simulink model "_Simulink_DualBoxcarAveragerFixedPoint"  (R2023b)
settings: Solver=FixedStepDiscrete  StartTime=0.0  StopTime=0.001  RelTol=1e-3
model workspace (MAT data in the model file):
  test = 0
undefined symbols (not defined in the file): a, b, c
libraries: hdlsllib x3, simulink x2, dspsrcs4 x1
settings Model: DataTypeOverride=Off  FPTShortcutValueString='{{},{''BaselineRun'',1,1,1,''BaselineRun'','''',{},''M'',''F'',''''},{''EmbeddedRun'',1,1,1,''EmbeddedRun'','''',{},''M'','''',''''},{''BaselineRun_5'',1,1,1,''BaselineRun_5'','''',{},''M'',''F'',''''}}'  Creator=max_d  LastModifiedBy=heyan
settings SolverCC: AlgebraicLoopSolver=TrustRegion  AutoInsertRateTranBlk=on
settings DataIOCC: LimitDataPoints=on  SaveOutput=off  SaveTime=off
settings OptimizationCC: BlockReduction=off  ConditionallyExecuteInputs=off  DefaultParameterBehavior=Inlined  InheritOutputTypeSmallerThanSingle=on  LifeSpan=inf
settings DebuggingCC: SignalRangeChecking=warning  AlgebraicLoopMsg=error  SingleTaskRateTransMsg=error  UnconnectedInputMsg=warning  UnconnectedOutputMsg=warning  UnconnectedLineMsg=warning  AllowSymbolicDim=off  StrictBusMsg=ErrorOnBusTreatedAsVector  SFUnexpectedBacktrackingDiag=warning  SFNoUnconditionalDefaultTransitionDiag=warning  SFExecutionAtInitializationDiag=none  ArithmeticOperatorsInVariantConditions=warning
settings HardwareCC: ProdBitPerPointer=32  ProdBitPerSizeT=32  ProdBitPerPtrDiffT=32  ProdLargestAtomicFloat=None  ProdIntDivRoundTo=Undefined  ProdEndianess=Unspecified  ProdWordSize=32  ProdHWDeviceType=ASIC/FPGA->ASIC/FPGA  ProdEqTarget=off
settings ModelReferenceCC: EnableRefExpFcnMdlSchedulingChecks=on
settings SFSimCC: SimUseLocalCustomCode=off  CustomCodeUndefinedFunction=UseInterfaceOnly
settings RTWCC: RTWUseLocalCustomCode=off  DLArmComputeVersion=19.05
settings CodeAppCC: StateflowObjectComments=on
settings GRTTargetCC: TargetLangStandard=C89/C90 (ANSI)
settings ConfigComp: CovScope=ReferencedModels  CovMetricSettings=dw  CovSaveCumulativeToWorkspaceVar=on  CovSaveSingleToWorkspaceVar=on  CovExternalEMLEnable=off  CovSFcnEnable=off

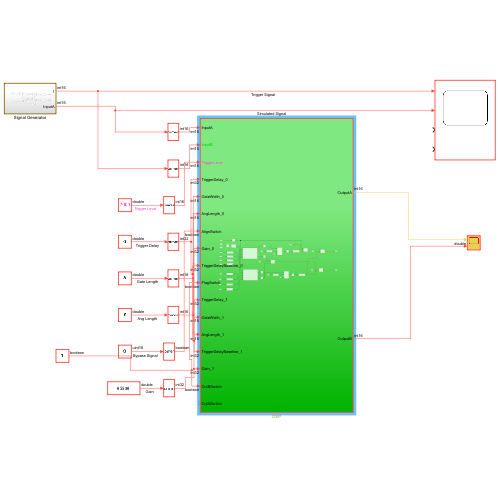
[thumbnail: Simulink's stored preview of the top-level diagram]
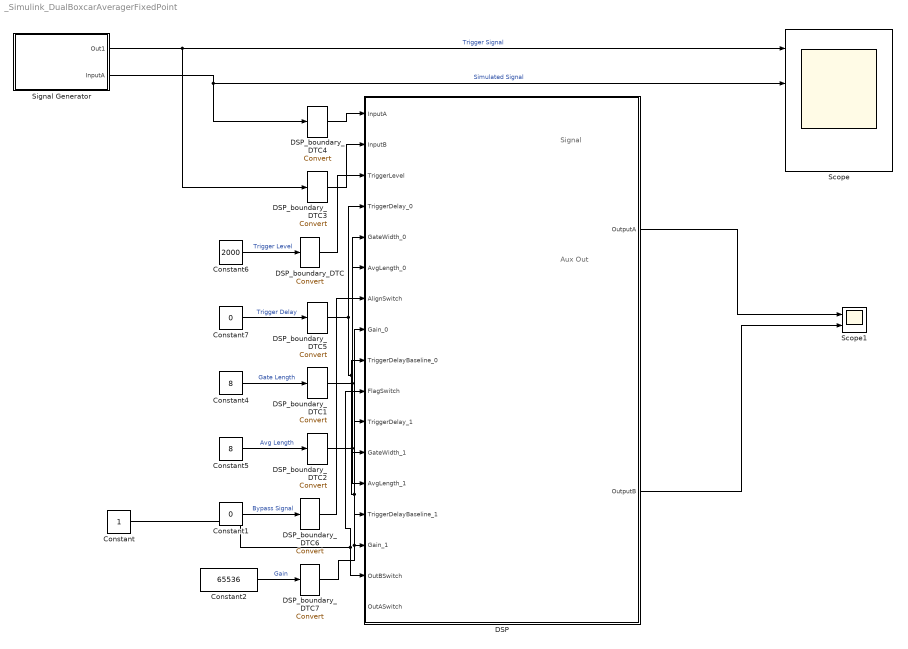
== system _Simulink_DualBoxcarAveragerFixedPoint ==
  note: Signal
  note: Aux Out
  Constant : Constant  OutDataTypeStr=boolean  SampleTime=1/312.5e6
  Constant1 : Constant  Value=0  OutDataTypeStr=fixdt(0,16,0)  SampleTime=1/312.5e6
  Constant2 : Constant  Value=65536  OutDataTypeStr=double  SampleTime=1/312.5e6
  Constant4 : Constant  Value=8  OutDataTypeStr=double  SampleTime=1/312.5e6
  Constant5 : Constant  Value=8  OutDataTypeStr=double  SampleTime=1/312.5e6
  Constant6 : Constant  Value=2000  OutDataTypeStr=double  SampleTime=1/312.5e6
  Constant7 : Constant  Value=0  OutDataTypeStr=double  SampleTime=1/312.5e6
  DSP : Subsystem
  DSP_boundary_DTC{,1..7} (8 alike) : DataTypeConversion
  Scope : Scope  NumInputPorts=4
  Scope1 : Scope  NumInputPorts=2
  Signal Generator : Subsystem
  wires:
  Constant2/1 -> DSP_boundary_DTC7/1  "Gain"
  Constant1/1 -> DSP_boundary_DTC6/1  "Bypass Signal"
  Constant5/1 -> DSP_boundary_DTC2/1  "Avg Length"
  Constant4/1 -> DSP_boundary_DTC1/1  "Gate Length"
  Constant7/1 -> DSP_boundary_DTC5/1  "Trigger Delay"
  Constant6/1 -> DSP_boundary_DTC/1  "Trigger Level"
  Signal Generator/1(Out1) -> DSP_boundary_DTC3/1, Scope/1  "Trigger Signal"
  Signal Generator/2(InputA) -> DSP_boundary_DTC4/1, Scope/2  "Simulated Signal"
  DSP_boundary_DTC/1 -> DSP/3(TriggerLevel)
  DSP_boundary_DTC1/1 -> DSP/12(GateWidth_1), DSP/5(GateWidth_0)
  DSP_boundary_DTC2/1 -> DSP/13(AvgLength_1), DSP/6(AvgLength_0)
  DSP_boundary_DTC3/1 -> DSP/2(InputB)
  DSP_boundary_DTC4/1 -> DSP/1(InputA)
  DSP_boundary_DTC5/1 -> DSP/9(TriggerDelayBaseline_0), DSP/14(TriggerDelayBaseline_1), DSP/11(TriggerDelay_1), DSP/4(TriggerDelay_0)
  DSP_boundary_DTC7/1 -> DSP/15(Gain_1), DSP/8(Gain_0)
  DSP_boundary_DTC6/1 -> DSP/7(AlignSwitch)
  Constant/1 -> DSP/16(OutBSwitch), DSP/10(FlagSwitch)
  DSP/1(OutputA) -> Scope1/1
  DSP/2(OutputB) -> Scope1/2

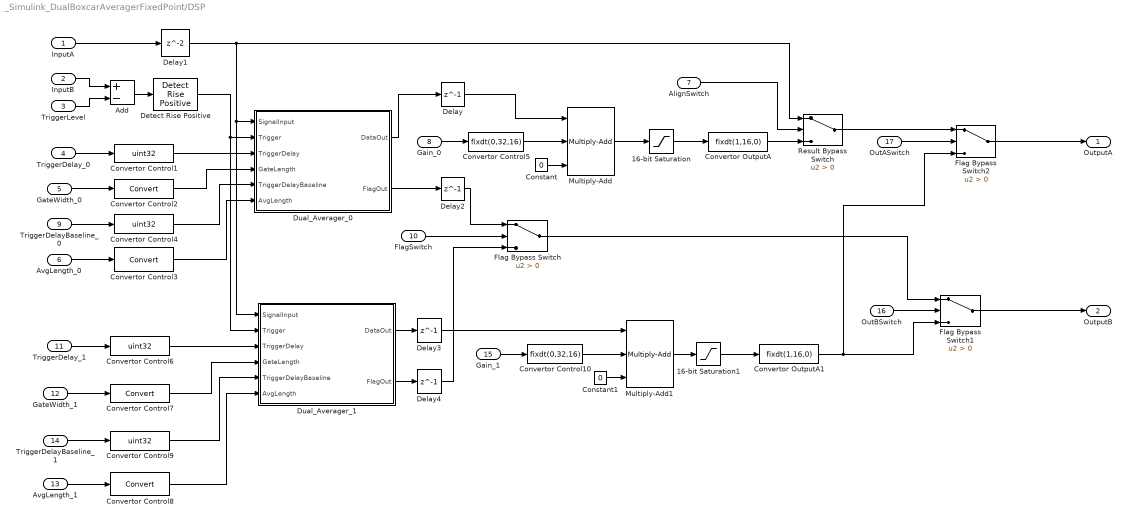
== system _Simulink_DualBoxcarAveragerFixedPoint/DSP ==
  InputA : Inport  OutDataTypeStr=fixdt(1,16,0)
  InputB : Inport  Port=2  OutDataTypeStr=fixdt(1,16,0)
  TriggerLevel : Inport  Port=3  OutDataTypeStr=fixdt(1,16,0)
  TriggerDelay_0 : Inport  Port=4  OutDataTypeStr=fixdt(1,32,0)
  GateWidth_0 : Inport  Port=5  OutDataTypeStr=fixdt(1,16,0)
  AvgLength_0 : Inport  Port=6  OutDataTypeStr=fixdt(1,16,0)
  AlignSwitch : Inport  Port=7  OutDataTypeStr=boolean
  Gain_0 : Inport  Port=8  OutDataTypeStr=fixdt(1,32,0)
  TriggerDelayBaseline_0 : Inport  Port=9  OutDataTypeStr=fixdt(1,32,0)
  FlagSwitch : Inport  Port=10  OutDataTypeStr=boolean
  TriggerDelay_1 : Inport  Port=11  OutDataTypeStr=fixdt(1,32,0)
  GateWidth_1 : Inport  Port=12  OutDataTypeStr=fixdt(1,16,0)
  AvgLength_1 : Inport  Port=13  OutDataTypeStr=fixdt(1,16,0)
  TriggerDelayBaseline_1 : Inport  Port=14  OutDataTypeStr=fixdt(1,32,0)
  Gain_1 : Inport  Port=15  OutDataTypeStr=fixdt(1,32,0)
  OutBSwitch : Inport  Port=16  OutDataTypeStr=boolean
  OutASwitch : Inport  Port=17  OutDataTypeStr=boolean
  16-bit Saturation : Saturate  UpperLimit=32767  LowerLimit=-32768
  16-bit Saturation1 : Saturate  UpperLimit=32767  LowerLimit=-32768
  Add : Sum  Inputs=+-  OutDataTypeStr=fixdt(1,17,0)
  Constant : Constant  Value=0  OutDataTypeStr=fixdt(0,1,0)  SampleTime=1/312.5e6
  Constant1 : Constant  Value=0  OutDataTypeStr=fixdt(0,1,0)  SampleTime=1/312.5e6
  Convertor Control{1,4,6,9} (4 alike) : DataTypeConversion  OutDataTypeStr=uint32  ConvertRealWorld=Stored Integer (SI)  SaturateOnIntegerOverflow=off  RndMeth=Floor
  Convertor Control10 : DataTypeConversion  OutDataTypeStr=fixdt(0,32,16)  ConvertRealWorld=Stored Integer (SI)  SaturateOnIntegerOverflow=off  RndMeth=Floor
  Convertor Control{2..3,7..8} (4 alike) : DataTypeConversion  ConvertRealWorld=Stored Integer (SI)  SaturateOnIntegerOverflow=off  RndMeth=Floor
  Convertor Control5 : DataTypeConversion  OutDataTypeStr=fixdt(0,32,16)  ConvertRealWorld=Stored Integer (SI)  SaturateOnIntegerOverflow=off  RndMeth=Floor
  Convertor OutputA : DataTypeConversion  OutDataTypeStr=fixdt(1,16,0)  SaturateOnIntegerOverflow=off  RndMeth=Floor
  Convertor OutputA1 : DataTypeConversion  OutDataTypeStr=fixdt(1,16,0)  SaturateOnIntegerOverflow=off  RndMeth=Floor
  Delay{,2..4} (4 alike) : Delay  DelayLength=1  InitialCondition=0  UseCircularBuffer=on
  Delay1 : Delay  InitialCondition=0
  Detect Rise Positive : hdlsllib/Logic and Bit Operations/Detect Rise Positive  vinit=0  OutDataTypeStr=boolean
  Dual_Averager_0 : Subsystem
  Dual_Averager_1 : Subsystem
  Flag Bypass Switch : Switch  Criteria=u2 > Threshold  SaturateOnIntegerOverflow=off  InputSameDT=off  OutDataTypeStr=Inherit: Same as first input
  Flag Bypass Switch1 : Switch  Criteria=u2 > Threshold  SaturateOnIntegerOverflow=off  InputSameDT=off  OutDataTypeStr=Inherit: Same as first input
  Flag Bypass Switch2 : Switch  Criteria=u2 > Threshold  SaturateOnIntegerOverflow=off  InputSameDT=off  OutDataTypeStr=Inherit: Same as first input
  Multiply-Add : hdlsllib/HDL Operations/Multiply-Add  Function=c+(a.*b)  datatype=Inherit: Inherit via internal rule  DoSatur=on  FMA=off
  Multiply-Add1 : hdlsllib/HDL Operations/Multiply-Add  Function=c+(a.*b)  datatype=Inherit: Inherit via internal rule  DoSatur=on  FMA=off
  Result Bypass Switch : Switch  Criteria=u2 > Threshold  OutDataTypeStr=fixdt(1,16,0)  SaturateOnIntegerOverflow=off  InputSameDT=off
  OutputA : Outport  OutDataTypeStr=fixdt(1,16,0)  VectorParamsAs1DForOutWhenUnconnected=off
  OutputB : Outport  Port=2  OutDataTypeStr=fixdt(1,16,0)  VectorParamsAs1DForOutWhenUnconnected=off
  wires:
  GateWidth_0/1 -> Convertor Control2/1
  Convertor OutputA/1 -> Result Bypass Switch/3
  Multiply-Add/1 -> 16-bit Saturation/1
  Constant/1 -> Multiply-Add/3
  TriggerLevel/1 -> Add/2
  Add/1 -> Detect Rise Positive/1
  Flag Bypass Switch/1 -> Flag Bypass Switch1/1
  16-bit Saturation/1 -> Convertor OutputA/1
  Gain_0/1 -> Convertor Control5/1
  Result Bypass Switch/1 -> Flag Bypass Switch2/1
  Convertor Control5/1 -> Multiply-Add/2
  InputA/1 -> Delay1/1
  AvgLength_0/1 -> Convertor Control3/1
  TriggerDelay_0/1 -> Convertor Control1/1
  InputB/1 -> Add/1
  TriggerDelayBaseline_0/1 -> Convertor Control4/1
  AlignSwitch/1 -> Result Bypass Switch/2
  FlagSwitch/1 -> Flag Bypass Switch/2
  TriggerDelay_1/1 -> Convertor Control6/1
  AvgLength_1/1 -> Convertor Control8/1
  GateWidth_1/1 -> Convertor Control7/1
  TriggerDelayBaseline_1/1 -> Convertor Control9/1
  Constant1/1 -> Multiply-Add1/3
  Multiply-Add1/1 -> 16-bit Saturation1/1
  Convertor Control10/1 -> Multiply-Add1/2
  16-bit Saturation1/1 -> Convertor OutputA1/1
  Gain_1/1 -> Convertor Control10/1
  OutBSwitch/1 -> Flag Bypass Switch1/2
  Convertor OutputA1/1 -> Flag Bypass Switch2/3, Flag Bypass Switch1/3
  Detect Rise Positive/1 -> Dual_Averager_1/2(Trigger), Dual_Averager_0/2(Trigger)
  Delay1/1 -> Dual_Averager_1/1(SignalInput), Dual_Averager_0/1(SignalInput), Result Bypass Switch/1
  Convertor Control1/1 -> Dual_Averager_0/3(TriggerDelay)
  Convertor Control4/1 -> Dual_Averager_0/5(TriggerDelayBaseline)
  Convertor Control2/1 -> Dual_Averager_0/4(GateLength)
  Convertor Control3/1 -> Dual_Averager_0/6(AvgLength)
  Dual_Averager_0/1(DataOut) -> Delay/1
  Dual_Averager_0/2(FlagOut) -> Delay2/1
  Convertor Control6/1 -> Dual_Averager_1/3(TriggerDelay)
  Convertor Control7/1 -> Dual_Averager_1/4(GateLength)
  Convertor Control9/1 -> Dual_Averager_1/5(TriggerDelayBaseline)
  Convertor Control8/1 -> Dual_Averager_1/6(AvgLength)
  Dual_Averager_1/2(FlagOut) -> Delay4/1
  Dual_Averager_1/1(DataOut) -> Delay3/1
  OutASwitch/1 -> Flag Bypass Switch2/2
  Flag Bypass Switch2/1 -> OutputA/1
  Flag Bypass Switch1/1 -> OutputB/1
  Delay/1 -> Multiply-Add/1
  Delay2/1 -> Flag Bypass Switch/1
  Delay3/1 -> Multiply-Add1/1
  Delay4/1 -> Flag Bypass Switch/3

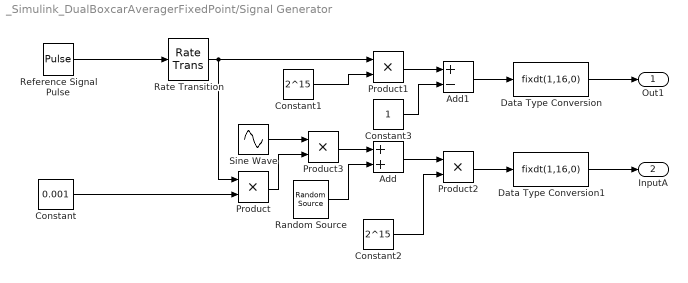
== system _Simulink_DualBoxcarAveragerFixedPoint/Signal Generator ==
  Add : Sum
  Add1 : Sum  Inputs=+-
  Constant : Constant  Value=0.001
  Constant1 : Constant  Value=2^15
  Constant2 : Constant  Value=2^15
  Constant3 : Constant
  Data Type Conversion : DataTypeConversion  OutDataTypeStr=fixdt(1,16,0)  SaturateOnIntegerOverflow=off  RndMeth=Floor
  Data Type Conversion1 : DataTypeConversion  OutDataTypeStr=fixdt(1,16,0)  SaturateOnIntegerOverflow=off  RndMeth=Floor
  Product{,1..3} (4 alike) : Product
  Random Source : dspsrcs4/Random Source  SrcType=Uniform  NormMethod=Ziggurat  CltLength=12  MinVal=-0.001  MaxVal=0.001  MeanVal=0  VarVal=1  RepMode=Not repeatable  rawSeed=1  IsInherit=off  SampMode=Discrete  SampTime=1/312.5e6  SampFrame=1  DataType=Double  OutComplex=Real  OutputFrames=off
  Rate Transition : RateTransition  OutPortSampleTime=1/312.5e6
  Reference Signal Pulse : DiscretePulseGenerator  PulseType=Time based  Period=100/(312.5e6)  PulseWidth=16
  Sine Wave : Sin  Amplitude=0.5  Bias=0.5  Frequency=2*pi*10e3  SampleTime=1/312.5e6
  Out1 : Outport  OutDataTypeStr=int16
  InputA : Outport  Port=2  OutDataTypeStr=int16
  wires:
  Data Type Conversion/1 -> Out1/1
  Reference Signal Pulse/1 -> Rate Transition/1
  Constant3/1 -> Add1/2
  Add1/1 -> Data Type Conversion/1
  Product1/1 -> Add1/1
  Product3/1 -> Add/1
  Random Source/1 -> Add/2
  Add/1 -> Product2/1
  Sine Wave/1 -> Product3/1
  Product2/1 -> Data Type Conversion1/1
  Constant2/1 -> Product2/2
  Constant/1 -> Product/2
  Product/1 -> Product3/2
  Constant1/1 -> Product1/2
  Data Type Conversion1/1 -> InputA/1
  Rate Transition/1 -> Product/1, Product1/1

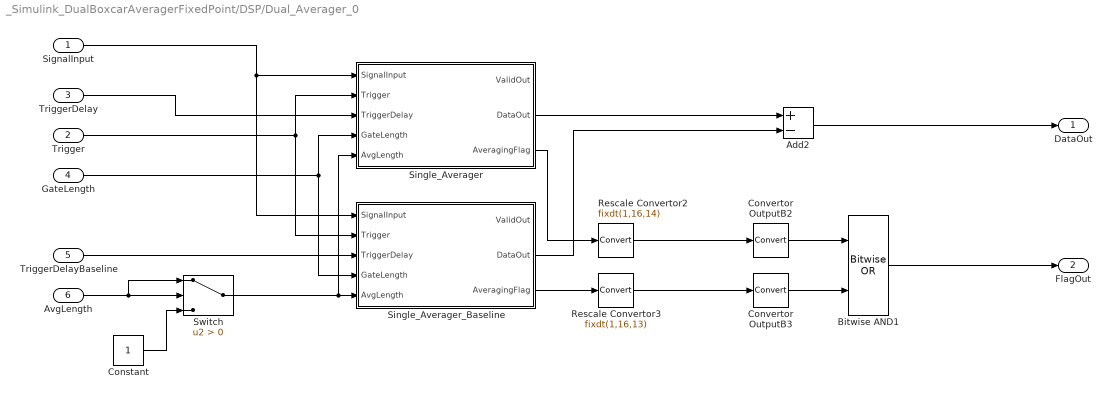
== system _Simulink_DualBoxcarAveragerFixedPoint/DSP/Dual_Averager_0 ==
  SignalInput : Inport
  Trigger : Inport  Port=2
  TriggerDelay : Inport  Port=3
  GateLength : Inport  Port=4
  TriggerDelayBaseline : Inport  Port=5
  AvgLength : Inport  Port=6
  Add2 : Sum  Inputs=+-
  Bitwise AND1 : simulink/Logic and Bit Operations/Bitwise Operator  logicop=OR  UseBitMask=off  NumInputPorts=2  BitMask=bin2dec('11011001')  BitMaskRealWorld=Stored Integer
      settings: LibrarySourceBlock=|
      | simulink/Quick Insert/Logic and Bit
      | Operations/Bitwise AND
  Constant : Constant  OutDataTypeStr=uint16  SampleTime=-1
  Convertor OutputB2 : DataTypeConversion  ConvertRealWorld=Stored Integer (SI)  SaturateOnIntegerOverflow=off  RndMeth=Floor
  Convertor OutputB3 : DataTypeConversion  ConvertRealWorld=Stored Integer (SI)  SaturateOnIntegerOverflow=off  RndMeth=Floor
  Rescale Convertor2 : DataTypeConversion  OutDataTypeStr=fixdt(1,16,14)  SaturateOnIntegerOverflow=off  RndMeth=Floor
  Rescale Convertor3 : DataTypeConversion  OutDataTypeStr=fixdt(1,16,13)  SaturateOnIntegerOverflow=off  RndMeth=Floor
  Single_Averager : Subsystem  TreatAsAtomicUnit=on
  Single_Averager_Baseline : Subsystem  TreatAsAtomicUnit=on
  Switch : Switch  Criteria=u2 > Threshold  SaturateOnIntegerOverflow=off  InputSameDT=off  OutDataTypeStr=Inherit: Same as first input
  DataOut : Outport
  FlagOut : Outport  Port=2
  wires:
  Single_Averager/3(AveragingFlag) -> Rescale Convertor2/1
  SignalInput/1 -> Single_Averager_Baseline/1(SignalInput), Single_Averager/1(SignalInput)
  Single_Averager_Baseline/2(DataOut) -> Add2/2
  GateLength/1 -> Single_Averager_Baseline/4(GateLength), Single_Averager/4(GateLength)
  Rescale Convertor3/1 -> Convertor OutputB3/1
  Single_Averager_Baseline/3(AveragingFlag) -> Rescale Convertor3/1
  Trigger/1 -> Single_Averager_Baseline/2(Trigger), Single_Averager/2(Trigger)
  Single_Averager/2(DataOut) -> Add2/1
  Rescale Convertor2/1 -> Convertor OutputB2/1
  Bitwise AND1/1 -> FlagOut/1
  Convertor OutputB2/1 -> Bitwise AND1/1
  Convertor OutputB3/1 -> Bitwise AND1/2
  TriggerDelayBaseline/1 -> Single_Averager_Baseline/3(TriggerDelay)
  Add2/1 -> DataOut/1
  TriggerDelay/1 -> Single_Averager/3(TriggerDelay)
  AvgLength/1 -> Switch/1, Switch/2
  Constant/1 -> Switch/3
  Switch/1 -> Single_Averager_Baseline/5(AvgLength), Single_Averager/5(AvgLength)

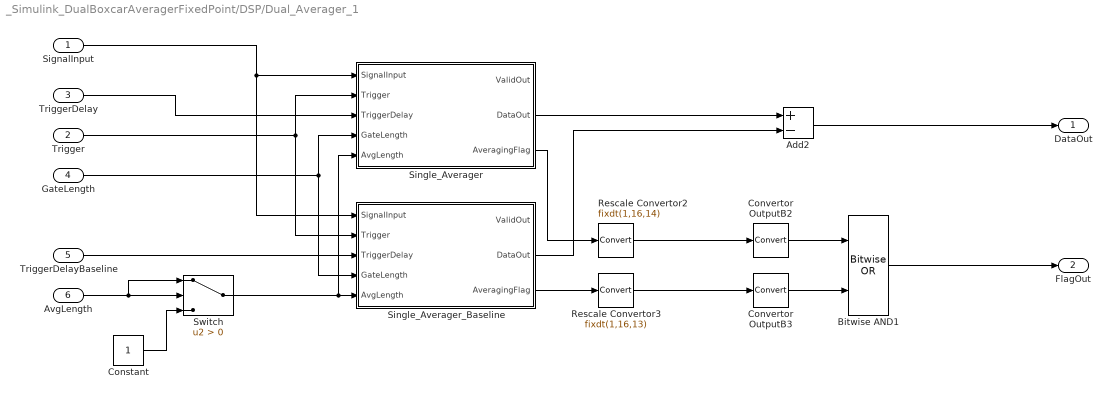
== system _Simulink_DualBoxcarAveragerFixedPoint/DSP/Dual_Averager_1 ==
  SignalInput : Inport
  Trigger : Inport  Port=2
  TriggerDelay : Inport  Port=3
  GateLength : Inport  Port=4
  TriggerDelayBaseline : Inport  Port=5
  AvgLength : Inport  Port=6
  Add2 : Sum  Inputs=+-
  Bitwise AND1 : simulink/Logic and Bit Operations/Bitwise Operator  logicop=OR  UseBitMask=off  NumInputPorts=2  BitMask=bin2dec('11011001')  BitMaskRealWorld=Stored Integer
      settings: LibrarySourceBlock=|
      | simulink/Quick Insert/Logic and Bit
      | Operations/Bitwise AND
  Constant : Constant  OutDataTypeStr=uint16  SampleTime=-1
  Convertor OutputB2 : DataTypeConversion  ConvertRealWorld=Stored Integer (SI)  SaturateOnIntegerOverflow=off  RndMeth=Floor
  Convertor OutputB3 : DataTypeConversion  ConvertRealWorld=Stored Integer (SI)  SaturateOnIntegerOverflow=off  RndMeth=Floor
  Rescale Convertor2 : DataTypeConversion  OutDataTypeStr=fixdt(1,16,14)  SaturateOnIntegerOverflow=off  RndMeth=Floor
  Rescale Convertor3 : DataTypeConversion  OutDataTypeStr=fixdt(1,16,13)  SaturateOnIntegerOverflow=off  RndMeth=Floor
  Single_Averager : Subsystem  TreatAsAtomicUnit=on
  Single_Averager_Baseline : Subsystem  TreatAsAtomicUnit=on
  Switch : Switch  Criteria=u2 > Threshold  SaturateOnIntegerOverflow=off  InputSameDT=off  OutDataTypeStr=Inherit: Same as first input
  DataOut : Outport
  FlagOut : Outport  Port=2
  wires:
  Single_Averager/3(AveragingFlag) -> Rescale Convertor2/1
  SignalInput/1 -> Single_Averager_Baseline/1(SignalInput), Single_Averager/1(SignalInput)
  Single_Averager_Baseline/2(DataOut) -> Add2/2
  GateLength/1 -> Single_Averager_Baseline/4(GateLength), Single_Averager/4(GateLength)
  Rescale Convertor3/1 -> Convertor OutputB3/1
  Single_Averager_Baseline/3(AveragingFlag) -> Rescale Convertor3/1
  Trigger/1 -> Single_Averager_Baseline/2(Trigger), Single_Averager/2(Trigger)
  Single_Averager/2(DataOut) -> Add2/1
  Rescale Convertor2/1 -> Convertor OutputB2/1
  Bitwise AND1/1 -> FlagOut/1
  Convertor OutputB2/1 -> Bitwise AND1/1
  Convertor OutputB3/1 -> Bitwise AND1/2
  TriggerDelayBaseline/1 -> Single_Averager_Baseline/3(TriggerDelay)
  Add2/1 -> DataOut/1
  TriggerDelay/1 -> Single_Averager/3(TriggerDelay)
  AvgLength/1 -> Switch/1, Switch/2
  Constant/1 -> Switch/3
  Switch/1 -> Single_Averager_Baseline/5(AvgLength), Single_Averager/5(AvgLength)

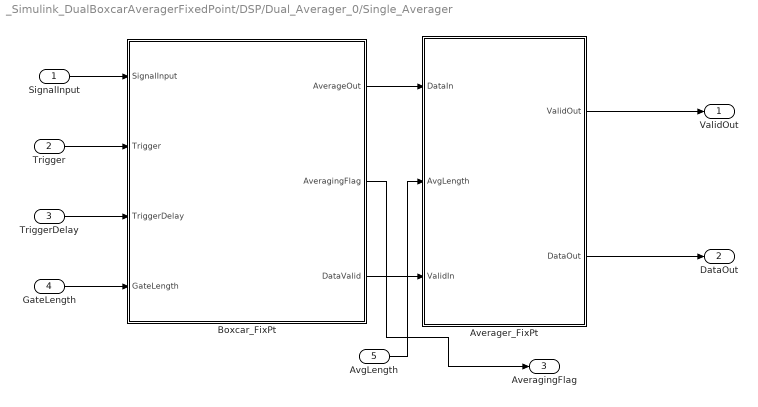
== system _Simulink_DualBoxcarAveragerFixedPoint/DSP/Dual_Averager_0/Single_Averager ==
  SignalInput : Inport
  Trigger : Inport  Port=2
  TriggerDelay : Inport  Port=3
  GateLength : Inport  Port=4
  AvgLength : Inport  Port=5
  Averager_FixPt : MATLAB Function  TreatAsAtomicUnit=on  VariantControl=(default)
  Boxcar_FixPt : MATLAB Function  TreatAsAtomicUnit=on  VariantControl=(default)
  ValidOut : Outport
  DataOut : Outport  Port=2
  AveragingFlag : Outport  Port=3
  wires:
  Boxcar_FixPt/1(AverageOut) -> Averager_FixPt/1(DataIn)
  Boxcar_FixPt/3(DataValid) -> Averager_FixPt/3(ValidIn)
  Averager_FixPt/1(ValidOut) -> ValidOut/1
  AvgLength/1 -> Averager_FixPt/2(AvgLength)
  Boxcar_FixPt/2(AveragingFlag) -> AveragingFlag/1
  TriggerDelay/1 -> Boxcar_FixPt/3(TriggerDelay)
  GateLength/1 -> Boxcar_FixPt/4(GateLength)
  SignalInput/1 -> Boxcar_FixPt/1(SignalInput)
  Averager_FixPt/2(DataOut) -> DataOut/1
  Trigger/1 -> Boxcar_FixPt/2(Trigger)

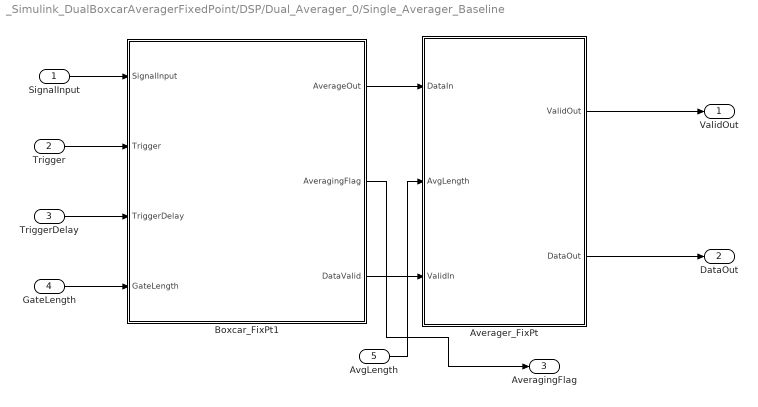
== system _Simulink_DualBoxcarAveragerFixedPoint/DSP/Dual_Averager_0/Single_Averager_Baseline ==
  SignalInput : Inport
  Trigger : Inport  Port=2
  TriggerDelay : Inport  Port=3
  GateLength : Inport  Port=4
  AvgLength : Inport  Port=5
  Averager_FixPt : MATLAB Function  TreatAsAtomicUnit=on  VariantControl=(default)
  Boxcar_FixPt1 : MATLAB Function  TreatAsAtomicUnit=on  VariantControl=(default)
  ValidOut : Outport
  DataOut : Outport  Port=2
  AveragingFlag : Outport  Port=3
  wires:
  Boxcar_FixPt1/1(AverageOut) -> Averager_FixPt/1(DataIn)
  Boxcar_FixPt1/3(DataValid) -> Averager_FixPt/3(ValidIn)
  Averager_FixPt/1(ValidOut) -> ValidOut/1
  AvgLength/1 -> Averager_FixPt/2(AvgLength)
  Boxcar_FixPt1/2(AveragingFlag) -> AveragingFlag/1
  TriggerDelay/1 -> Boxcar_FixPt1/3(TriggerDelay)
  GateLength/1 -> Boxcar_FixPt1/4(GateLength)
  SignalInput/1 -> Boxcar_FixPt1/1(SignalInput)
  Averager_FixPt/2(DataOut) -> DataOut/1
  Trigger/1 -> Boxcar_FixPt1/2(Trigger)

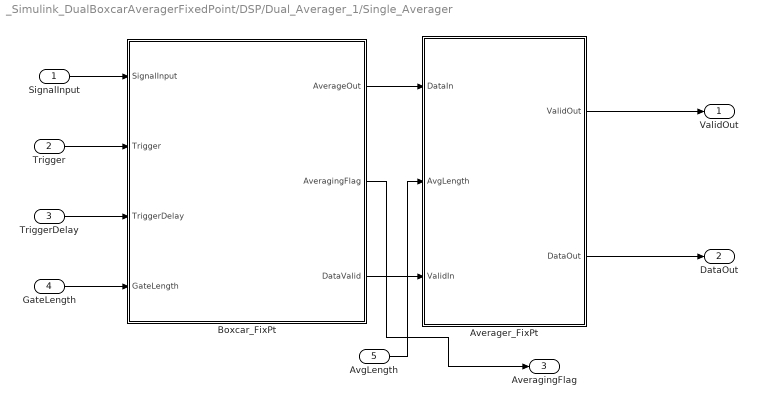
== system _Simulink_DualBoxcarAveragerFixedPoint/DSP/Dual_Averager_1/Single_Averager ==
  SignalInput : Inport
  Trigger : Inport  Port=2
  TriggerDelay : Inport  Port=3
  GateLength : Inport  Port=4
  AvgLength : Inport  Port=5
  Averager_FixPt : MATLAB Function  TreatAsAtomicUnit=on  VariantControl=(default)
  Boxcar_FixPt : MATLAB Function  TreatAsAtomicUnit=on  VariantControl=(default)
  ValidOut : Outport
  DataOut : Outport  Port=2
  AveragingFlag : Outport  Port=3
  wires:
  Boxcar_FixPt/1(AverageOut) -> Averager_FixPt/1(DataIn)
  Boxcar_FixPt/3(DataValid) -> Averager_FixPt/3(ValidIn)
  Averager_FixPt/1(ValidOut) -> ValidOut/1
  AvgLength/1 -> Averager_FixPt/2(AvgLength)
  Boxcar_FixPt/2(AveragingFlag) -> AveragingFlag/1
  TriggerDelay/1 -> Boxcar_FixPt/3(TriggerDelay)
  GateLength/1 -> Boxcar_FixPt/4(GateLength)
  SignalInput/1 -> Boxcar_FixPt/1(SignalInput)
  Averager_FixPt/2(DataOut) -> DataOut/1
  Trigger/1 -> Boxcar_FixPt/2(Trigger)

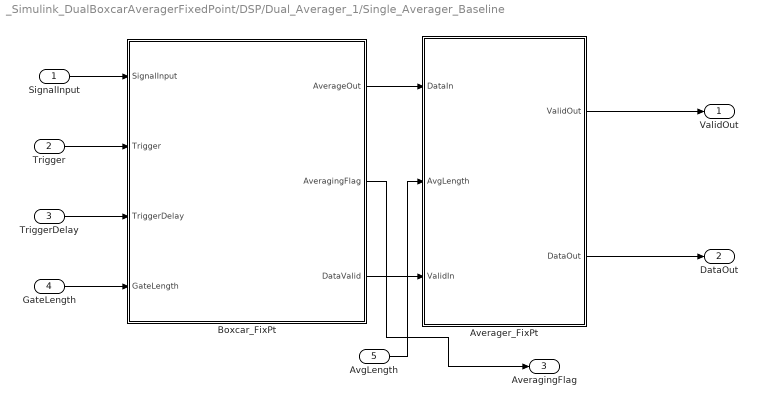
== system _Simulink_DualBoxcarAveragerFixedPoint/DSP/Dual_Averager_1/Single_Averager_Baseline ==
  SignalInput : Inport
  Trigger : Inport  Port=2
  TriggerDelay : Inport  Port=3
  GateLength : Inport  Port=4
  AvgLength : Inport  Port=5
  Averager_FixPt : MATLAB Function  TreatAsAtomicUnit=on  VariantControl=(default)
  Boxcar_FixPt : MATLAB Function  TreatAsAtomicUnit=on  VariantControl=(default)
  ValidOut : Outport
  DataOut : Outport  Port=2
  AveragingFlag : Outport  Port=3
  wires:
  Boxcar_FixPt/1(AverageOut) -> Averager_FixPt/1(DataIn)
  Boxcar_FixPt/3(DataValid) -> Averager_FixPt/3(ValidIn)
  Averager_FixPt/1(ValidOut) -> ValidOut/1
  AvgLength/1 -> Averager_FixPt/2(AvgLength)
  Boxcar_FixPt/2(AveragingFlag) -> AveragingFlag/1
  TriggerDelay/1 -> Boxcar_FixPt/3(TriggerDelay)
  GateLength/1 -> Boxcar_FixPt/4(GateLength)
  SignalInput/1 -> Boxcar_FixPt/1(SignalInput)
  Averager_FixPt/2(DataOut) -> DataOut/1
  Trigger/1 -> Boxcar_FixPt/2(Trigger)

== matlab function _Simulink_DualBoxcarAveragerFixedPoint/DSP/Dual_Averager_0/Single_Averager_Baseline/Averager_FixPt ==
  settings: fimath=fimath('RoundingMethod', 'Floor', 'OverflowAction', 'Wrap', 'ProductMode', 'FullPrecision', 'MaxProductWordLength', 128, 'SumMode', 'FullPrecision', 'MaxSumWordLength', 128)
  data: DataIn input fixdt(1,32,0); AvgLength input uint16; ValidIn input fixdt(0,1,0); ValidOut output fixdt(0,1,0); DataOut output fixdt(1,48,0)
%auto-generated
function [ValidOut,DataOut] = Average_fixpt(DataIn,AvgLength,ValidIn)
%#codegen

fm = get_fimath();
AvgLength = fi(AvgLength, 0, 16, 0, fm);
DataIn = fi(DataIn, 1, 32, 0, fm);
ValidIn = fi(ValidIn, 0, 1, 0, fm);

persistent AvgOut;
if isempty(AvgOut)
    AvgOut = fi(0, 1, 48, 0, fm);
end

persistent DataOutReg;
if isempty(DataOutReg)
    DataOutReg = fi(0, 1, 48, 0, fm);
end

persistent ValidOutReg;
if isempty(ValidOutReg)
    ValidOutReg = fi(0, 0, 1, 0, fm);
end

persistent cnt1;
if isempty(cnt1)
    cnt1 = fi(0, 0, 16, 0, fm);
end


S1 = fi(0, 0, 1, 0, fm); %Waiting for trigger
S2 = fi(1, 0, 1, 0, fm);

persistent current_state;
if isempty(current_state)
    current_state = fi(S1, 0, 1, 0, fm);   
end

switch(current_state)

    case S1
        ValidOutReg(:) = 0;
        if ValidIn == fi(1, 0, 1, 0, fm)
            current_state(:) = S2;
            cnt1(:) = fi_signed(AvgLength)-fi(1, 0, 1, 0, fm);
            AvgOut(:) = DataIn;
        else
            current_state(:) = S1;
        end

    case S2

        if ValidIn == fi(1, 0, 1, 0, fm)
            AvgOut(:) = AvgOut+DataIn;
            cnt1(:) = fi_signed(cnt1)-fi(1, 0, 1, 0, fm);
        end
        if cnt1 == fi(0, 0, 1, 0, fm)
            DataOutReg(:) = AvgOut;
            ValidOutReg(:) = 1;
            current_state(:) = S1;
        end

end

DataOut = fi(DataOutReg, 1, 48, 0, fm);
ValidOut = fi(ValidOutReg, 0, 1, 0, fm);

end



function y = fi_signed(a)
    coder.inline( 'always' );
    if isfi( a ) && ~(issigned( a ))
        nt = numerictype( a );
        new_nt = numerictype( 1, nt.WordLength + 1, nt.FractionLength );
        y = fi( a, new_nt, fimath( a ) );
    else
        y = a;
    end
end

function fm = get_fimath()
	fm = fimath('RoundingMethod', 'Floor',...
	     'OverflowAction', 'Wrap',...
	     'ProductMode','FullPrecision',...
	     'MaxProductWordLength', 128,...
	     'SumMode','FullPrecision',...
	     'MaxSumWordLength', 128);
end

== matlab function _Simulink_DualBoxcarAveragerFixedPoint/DSP/Dual_Averager_0/Single_Averager/Averager_FixPt ==
  settings: fimath=fimath('RoundingMethod', 'Floor', 'OverflowAction', 'Wrap', 'ProductMode', 'FullPrecision', 'MaxProductWordLength', 128, 'SumMode', 'FullPrecision', 'MaxSumWordLength', 128)
  data: DataIn input fixdt(1,32,0); AvgLength input uint16; ValidIn input fixdt(0,1,0); ValidOut output fixdt(0,1,0); DataOut output fixdt(1,48,0)
%auto-generated
function [ValidOut,DataOut] = Average_fixpt(DataIn,AvgLength,ValidIn)
%#codegen

fm = get_fimath();
AvgLength = fi(AvgLength, 0, 16, 0, fm);
DataIn = fi(DataIn, 1, 32, 0, fm);
ValidIn = fi(ValidIn, 0, 1, 0, fm);

persistent AvgOut;
if isempty(AvgOut)
    AvgOut = fi(0, 1, 48, 0, fm);
end

persistent DataOutReg;
if isempty(DataOutReg)
    DataOutReg = fi(0, 1, 48, 0, fm);
end

persistent ValidOutReg;
if isempty(ValidOutReg)
    ValidOutReg = fi(0, 0, 1, 0, fm);
end

persistent cnt1;
if isempty(cnt1)
    cnt1 = fi(0, 0, 16, 0, fm);
end


S1 = fi(0, 0, 1, 0, fm); %Waiting for trigger
S2 = fi(1, 0, 1, 0, fm);

persistent current_state;
if isempty(current_state)
    current_state = fi(S1, 0, 1, 0, fm);   
end

switch(current_state)

    case S1
        ValidOutReg(:) = 0;
        if ValidIn == fi(1, 0, 1, 0, fm)
            current_state(:) = S2;
            cnt1(:) = fi_signed(AvgLength)-fi(1, 0, 1, 0, fm);
            AvgOut(:) = DataIn;
        else
            current_state(:) = S1;
        end

    case S2

        if ValidIn == fi(1, 0, 1, 0, fm)
            AvgOut(:) = AvgOut+DataIn;
            cnt1(:) = fi_signed(cnt1)-fi(1, 0, 1, 0, fm);
        end
        if cnt1 == fi(0, 0, 1, 0, fm)
            DataOutReg(:) = AvgOut;
            ValidOutReg(:) = 1;
            current_state(:) = S1;
        end

end

DataOut = fi(DataOutReg, 1, 48, 0, fm);
ValidOut = fi(ValidOutReg, 0, 1, 0, fm);

end



function y = fi_signed(a)
    coder.inline( 'always' );
    if isfi( a ) && ~(issigned( a ))
        nt = numerictype( a );
        new_nt = numerictype( 1, nt.WordLength + 1, nt.FractionLength );
        y = fi( a, new_nt, fimath( a ) );
    else
        y = a;
    end
end

function fm = get_fimath()
	fm = fimath('RoundingMethod', 'Floor',...
	     'OverflowAction', 'Wrap',...
	     'ProductMode','FullPrecision',...
	     'MaxProductWordLength', 128,...
	     'SumMode','FullPrecision',...
	     'MaxSumWordLength', 128);
end

== matlab function _Simulink_DualBoxcarAveragerFixedPoint/DSP/Dual_Averager_1/Single_Averager/Boxcar_FixPt ==
  settings: fimath=fimath('RoundingMethod', 'Floor', 'OverflowAction', 'Wrap', 'ProductMode', 'FullPrecision', 'MaxProductWordLength', 128, 'SumMode', 'FullPrecision', 'MaxSumWordLength', 128)
  data: SignalInput input int16 size=1; AverageOut output fixdt(1,32,0) size=1; Trigger input boolean size=1; TriggerDelay input uint32 size=1; GateLength input uint16; AveragingFlag output fixdt(0,1,0); DataValid output fixdt(0,1,0)
%auto-generated
%#codegen
function [AverageOut,AveragingFlag,DataValid] = Boxcar_fixpt(SignalInput, Trigger, TriggerDelay, GateLength)

fm = get_fimath();
GateLength = fi(GateLength, 0, 16, 0, fm);
SignalInput = fi(SignalInput, 1, 16, 0, fm);
TriggerDelay = fi(TriggerDelay, 0, 32, 0, fm);

persistent AvgOut;
if isempty(AvgOut)
    AvgOut = fi(0, 1, 32, 0, fm);
end


persistent cnt1;
if isempty(cnt1)
    cnt1 = fi(0, 0, 32, 0, fm);
end

persistent cnt2;
if isempty(cnt2)
    cnt2 = fi(0, 0, 16, 0, fm);
end


persistent AvgFlag;
if isempty(AvgFlag)
    AvgFlag = fi(0, 0, 1, 0, fm);
end

persistent DValid;
if isempty(DValid)
    DValid = fi(0, 0, 1, 0, fm);
end

S1 = fi(0, 0, 2, 0, fm); %Waiting for trigger
S2 = fi(1, 0, 2, 0, fm);
S3 = fi(2, 0, 2, 0, fm);

persistent current_state;
if isempty(current_state)
    current_state = fi(S1, 0, 2, 0, fm);   
end

switch(current_state)

    case S1
        DValid(:) = 0;
        AvgFlag(:) = 0;
        if Trigger == 1
            current_state(:) = S2;
            cnt1(:) = TriggerDelay;
        else
            current_state(:) = S1;
        end

    case S2

        if cnt1 == fi(0, 0, 1, 0, fm)
            current_state(:) = S3;
            cnt2(:) = GateLength;
            AvgOut(:) = 0;
        else
            cnt1(:) = fi_signed(cnt1)-fi(1, 0, 1, 0, fm);
        end

    case S3
        if cnt2 == fi(0, 0, 1, 0, fm)
            current_state(:) = S1;
            DValid(:) = 0;
        else
            AvgOut(:) = AvgOut + SignalInput;
            AvgFlag(:) = 1;
            cnt2(:) = fi_signed(cnt2)-fi(1, 0, 1, 0, fm);
            if cnt2 == fi(0, 0, 1, 0, fm)
                DValid(:) = 1;
                current_state(:) = S1;
            end 
        end

end

AverageOut = fi(AvgOut, 1, 32, 0, fm);
DataValid = fi(DValid, 0, 1, 0, fm);
AveragingFlag = fi(AvgFlag, 0, 1, 0, fm);



end



function y = fi_signed(a)
    coder.inline( 'always' );
    if isfi( a ) && ~(issigned( a ))
        nt = numerictype( a );
        new_nt = numerictype( 1, nt.WordLength + 1, nt.FractionLength );
        y = fi( a, new_nt, fimath( a ) );
    else
        y = a;
    end
end

function fm = get_fimath()
	fm = fimath('RoundingMethod', 'Floor',...
	     'OverflowAction', 'Wrap',...
	     'ProductMode','FullPrecision',...
	     'MaxProductWordLength', 128,...
	     'SumMode','FullPrecision',...
	     'MaxSumWordLength', 128);
end

== matlab function _Simulink_DualBoxcarAveragerFixedPoint/DSP/Dual_Averager_0/Single_Averager/Boxcar_FixPt ==
  settings: fimath=fimath('RoundingMethod', 'Floor', 'OverflowAction', 'Wrap', 'ProductMode', 'FullPrecision', 'MaxProductWordLength', 128, 'SumMode', 'FullPrecision', 'MaxSumWordLength', 128)
  data: SignalInput input int16 size=1; AverageOut output fixdt(1,32,0) size=1; Trigger input boolean size=1; TriggerDelay input uint32 size=1; GateLength input uint16; AveragingFlag output fixdt(0,1,0); DataValid output fixdt(0,1,0)
%auto-generated
%#codegen
function [AverageOut,AveragingFlag,DataValid] = Boxcar_fixpt(SignalInput, Trigger, TriggerDelay, GateLength)

fm = get_fimath();
GateLength = fi(GateLength, 0, 16, 0, fm);
SignalInput = fi(SignalInput, 1, 16, 0, fm);
TriggerDelay = fi(TriggerDelay, 0, 32, 0, fm);

persistent AvgOut;
if isempty(AvgOut)
    AvgOut = fi(0, 1, 32, 0, fm);
end


persistent cnt1;
if isempty(cnt1)
    cnt1 = fi(0, 0, 32, 0, fm);
end

persistent cnt2;
if isempty(cnt2)
    cnt2 = fi(0, 0, 16, 0, fm);
end


persistent AvgFlag;
if isempty(AvgFlag)
    AvgFlag = fi(0, 0, 1, 0, fm);
end

persistent DValid;
if isempty(DValid)
    DValid = fi(0, 0, 1, 0, fm);
end

S1 = fi(0, 0, 2, 0, fm); %Waiting for trigger
S2 = fi(1, 0, 2, 0, fm);
S3 = fi(2, 0, 2, 0, fm);

persistent current_state;
if isempty(current_state)
    current_state = fi(S1, 0, 2, 0, fm);   
end

switch(current_state)

    case S1
        DValid(:) = 0;
        AvgFlag(:) = 0;
        if Trigger == 1
            current_state(:) = S2;
            cnt1(:) = TriggerDelay;
        else
            current_state(:) = S1;
        end

    case S2

        if cnt1 == fi(0, 0, 1, 0, fm)
            current_state(:) = S3;
            cnt2(:) = GateLength;
            AvgOut(:) = 0;
        else
            cnt1(:) = fi_signed(cnt1)-fi(1, 0, 1, 0, fm);
        end

    case S3
        if cnt2 == fi(0, 0, 1, 0, fm)
            current_state(:) = S1;
            DValid(:) = 0;
        else
            AvgOut(:) = AvgOut + SignalInput;
            AvgFlag(:) = 1;
            cnt2(:) = fi_signed(cnt2)-fi(1, 0, 1, 0, fm);
            if cnt2 == fi(0, 0, 1, 0, fm)
                DValid(:) = 1;
                current_state(:) = S1;
            end 
        end

end

AverageOut = fi(AvgOut, 1, 32, 0, fm);
DataValid = fi(DValid, 0, 1, 0, fm);
AveragingFlag = fi(AvgFlag, 0, 1, 0, fm);



end



function y = fi_signed(a)
    coder.inline( 'always' );
    if isfi( a ) && ~(issigned( a ))
        nt = numerictype( a );
        new_nt = numerictype( 1, nt.WordLength + 1, nt.FractionLength );
        y = fi( a, new_nt, fimath( a ) );
    else
        y = a;
    end
end

function fm = get_fimath()
	fm = fimath('RoundingMethod', 'Floor',...
	     'OverflowAction', 'Wrap',...
	     'ProductMode','FullPrecision',...
	     'MaxProductWordLength', 128,...
	     'SumMode','FullPrecision',...
	     'MaxSumWordLength', 128);
end

== matlab function _Simulink_DualBoxcarAveragerFixedPoint/DSP/Dual_Averager_1/Single_Averager/Averager_FixPt ==
  settings: fimath=fimath('RoundingMethod', 'Floor', 'OverflowAction', 'Wrap', 'ProductMode', 'FullPrecision', 'MaxProductWordLength', 128, 'SumMode', 'FullPrecision', 'MaxSumWordLength', 128)
  data: DataIn input fixdt(1,32,0); AvgLength input uint16; ValidIn input fixdt(0,1,0); ValidOut output fixdt(0,1,0); DataOut output fixdt(1,48,0)
%auto-generated
function [ValidOut,DataOut] = Average_fixpt(DataIn,AvgLength,ValidIn)
%#codegen

fm = get_fimath();
AvgLength = fi(AvgLength, 0, 16, 0, fm);
DataIn = fi(DataIn, 1, 32, 0, fm);
ValidIn = fi(ValidIn, 0, 1, 0, fm);

persistent AvgOut;
if isempty(AvgOut)
    AvgOut = fi(0, 1, 48, 0, fm);
end

persistent DataOutReg;
if isempty(DataOutReg)
    DataOutReg = fi(0, 1, 48, 0, fm);
end

persistent ValidOutReg;
if isempty(ValidOutReg)
    ValidOutReg = fi(0, 0, 1, 0, fm);
end

persistent cnt1;
if isempty(cnt1)
    cnt1 = fi(0, 0, 16, 0, fm);
end


S1 = fi(0, 0, 1, 0, fm); %Waiting for trigger
S2 = fi(1, 0, 1, 0, fm);

persistent current_state;
if isempty(current_state)
    current_state = fi(S1, 0, 1, 0, fm);   
end

switch(current_state)

    case S1
        ValidOutReg(:) = 0;
        if ValidIn == fi(1, 0, 1, 0, fm)
            current_state(:) = S2;
            cnt1(:) = fi_signed(AvgLength)-fi(1, 0, 1, 0, fm);
            AvgOut(:) = DataIn;
        else
            current_state(:) = S1;
        end

    case S2

        if ValidIn == fi(1, 0, 1, 0, fm)
            AvgOut(:) = AvgOut+DataIn;
            cnt1(:) = fi_signed(cnt1)-fi(1, 0, 1, 0, fm);
        end
        if cnt1 == fi(0, 0, 1, 0, fm)
            DataOutReg(:) = AvgOut;
            ValidOutReg(:) = 1;
            current_state(:) = S1;
        end

end

DataOut = fi(DataOutReg, 1, 48, 0, fm);
ValidOut = fi(ValidOutReg, 0, 1, 0, fm);

end



function y = fi_signed(a)
    coder.inline( 'always' );
    if isfi( a ) && ~(issigned( a ))
        nt = numerictype( a );
        new_nt = numerictype( 1, nt.WordLength + 1, nt.FractionLength );
        y = fi( a, new_nt, fimath( a ) );
    else
        y = a;
    end
end

function fm = get_fimath()
	fm = fimath('RoundingMethod', 'Floor',...
	     'OverflowAction', 'Wrap',...
	     'ProductMode','FullPrecision',...
	     'MaxProductWordLength', 128,...
	     'SumMode','FullPrecision',...
	     'MaxSumWordLength', 128);
end

== matlab function _Simulink_DualBoxcarAveragerFixedPoint/DSP/Dual_Averager_1/Single_Averager_Baseline/Boxcar_FixPt ==
  settings: fimath=fimath('RoundingMethod', 'Floor', 'OverflowAction', 'Wrap', 'ProductMode', 'FullPrecision', 'MaxProductWordLength', 128, 'SumMode', 'FullPrecision', 'MaxSumWordLength', 128)
  data: SignalInput input int16 size=1; AverageOut output fixdt(1,32,0) size=1; Trigger input boolean size=1; TriggerDelay input uint32 size=1; GateLength input uint16; AveragingFlag output fixdt(0,1,0); DataValid output fixdt(0,1,0)
%auto-generated
%#codegen
function [AverageOut,AveragingFlag,DataValid] = Boxcar_fixpt(SignalInput, Trigger, TriggerDelay, GateLength)

fm = get_fimath();
GateLength = fi(GateLength, 0, 16, 0, fm);
SignalInput = fi(SignalInput, 1, 16, 0, fm);
TriggerDelay = fi(TriggerDelay, 0, 32, 0, fm);

persistent AvgOut;
if isempty(AvgOut)
    AvgOut = fi(0, 1, 32, 0, fm);
end


persistent cnt1;
if isempty(cnt1)
    cnt1 = fi(0, 0, 32, 0, fm);
end

persistent cnt2;
if isempty(cnt2)
    cnt2 = fi(0, 0, 16, 0, fm);
end


persistent AvgFlag;
if isempty(AvgFlag)
    AvgFlag = fi(0, 0, 1, 0, fm);
end

persistent DValid;
if isempty(DValid)
    DValid = fi(0, 0, 1, 0, fm);
end

S1 = fi(0, 0, 2, 0, fm); %Waiting for trigger
S2 = fi(1, 0, 2, 0, fm);
S3 = fi(2, 0, 2, 0, fm);

persistent current_state;
if isempty(current_state)
    current_state = fi(S1, 0, 2, 0, fm);   
end

switch(current_state)

    case S1
        DValid(:) = 0;
        AvgFlag(:) = 0;
        if Trigger == 1
            current_state(:) = S2;
            cnt1(:) = TriggerDelay;
        else
            current_state(:) = S1;
        end

    case S2

        if cnt1 == fi(0, 0, 1, 0, fm)
            current_state(:) = S3;
            cnt2(:) = GateLength;
            AvgOut(:) = 0;
        else
            cnt1(:) = fi_signed(cnt1)-fi(1, 0, 1, 0, fm);
        end

    case S3
        if cnt2 == fi(0, 0, 1, 0, fm)
            current_state(:) = S1;
            DValid(:) = 0;
        else
            AvgOut(:) = AvgOut + SignalInput;
            AvgFlag(:) = 1;
            cnt2(:) = fi_signed(cnt2)-fi(1, 0, 1, 0, fm);
            if cnt2 == fi(0, 0, 1, 0, fm)
                DValid(:) = 1;
                current_state(:) = S1;
            end 
        end

end

AverageOut = fi(AvgOut, 1, 32, 0, fm);
DataValid = fi(DValid, 0, 1, 0, fm);
AveragingFlag = fi(AvgFlag, 0, 1, 0, fm);



end



function y = fi_signed(a)
    coder.inline( 'always' );
    if isfi( a ) && ~(issigned( a ))
        nt = numerictype( a );
        new_nt = numerictype( 1, nt.WordLength + 1, nt.FractionLength );
        y = fi( a, new_nt, fimath( a ) );
    else
        y = a;
    end
end

function fm = get_fimath()
	fm = fimath('RoundingMethod', 'Floor',...
	     'OverflowAction', 'Wrap',...
	     'ProductMode','FullPrecision',...
	     'MaxProductWordLength', 128,...
	     'SumMode','FullPrecision',...
	     'MaxSumWordLength', 128);
end

== matlab function _Simulink_DualBoxcarAveragerFixedPoint/DSP/Dual_Averager_1/Single_Averager_Baseline/Averager_FixPt ==
  settings: fimath=fimath('RoundingMethod', 'Floor', 'OverflowAction', 'Wrap', 'ProductMode', 'FullPrecision', 'MaxProductWordLength', 128, 'SumMode', 'FullPrecision', 'MaxSumWordLength', 128)
  data: DataIn input fixdt(1,32,0); AvgLength input uint16; ValidIn input fixdt(0,1,0); ValidOut output fixdt(0,1,0); DataOut output fixdt(1,48,0)
%auto-generated
function [ValidOut,DataOut] = Average_fixpt(DataIn,AvgLength,ValidIn)
%#codegen

fm = get_fimath();
AvgLength = fi(AvgLength, 0, 16, 0, fm);
DataIn = fi(DataIn, 1, 32, 0, fm);
ValidIn = fi(ValidIn, 0, 1, 0, fm);

persistent AvgOut;
if isempty(AvgOut)
    AvgOut = fi(0, 1, 48, 0, fm);
end

persistent DataOutReg;
if isempty(DataOutReg)
    DataOutReg = fi(0, 1, 48, 0, fm);
end

persistent ValidOutReg;
if isempty(ValidOutReg)
    ValidOutReg = fi(0, 0, 1, 0, fm);
end

persistent cnt1;
if isempty(cnt1)
    cnt1 = fi(0, 0, 16, 0, fm);
end


S1 = fi(0, 0, 1, 0, fm); %Waiting for trigger
S2 = fi(1, 0, 1, 0, fm);

persistent current_state;
if isempty(current_state)
    current_state = fi(S1, 0, 1, 0, fm);   
end

switch(current_state)

    case S1
        ValidOutReg(:) = 0;
        if ValidIn == fi(1, 0, 1, 0, fm)
            current_state(:) = S2;
            cnt1(:) = fi_signed(AvgLength)-fi(1, 0, 1, 0, fm);
            AvgOut(:) = DataIn;
        else
            current_state(:) = S1;
        end

    case S2

        if ValidIn == fi(1, 0, 1, 0, fm)
            AvgOut(:) = AvgOut+DataIn;
            cnt1(:) = fi_signed(cnt1)-fi(1, 0, 1, 0, fm);
        end
        if cnt1 == fi(0, 0, 1, 0, fm)
            DataOutReg(:) = AvgOut;
            ValidOutReg(:) = 1;
            current_state(:) = S1;
        end

end

DataOut = fi(DataOutReg, 1, 48, 0, fm);
ValidOut = fi(ValidOutReg, 0, 1, 0, fm);

end



function y = fi_signed(a)
    coder.inline( 'always' );
    if isfi( a ) && ~(issigned( a ))
        nt = numerictype( a );
        new_nt = numerictype( 1, nt.WordLength + 1, nt.FractionLength );
        y = fi( a, new_nt, fimath( a ) );
    else
        y = a;
    end
end

function fm = get_fimath()
	fm = fimath('RoundingMethod', 'Floor',...
	     'OverflowAction', 'Wrap',...
	     'ProductMode','FullPrecision',...
	     'MaxProductWordLength', 128,...
	     'SumMode','FullPrecision',...
	     'MaxSumWordLength', 128);
end

== matlab function _Simulink_DualBoxcarAveragerFixedPoint/DSP/Dual_Averager_0/Single_Averager_Baseline/Boxcar_FixPt1 ==
  settings: fimath=fimath('RoundingMethod', 'Floor', 'OverflowAction', 'Wrap', 'ProductMode', 'FullPrecision', 'MaxProductWordLength', 128, 'SumMode', 'FullPrecision', 'MaxSumWordLength', 128)
  data: SignalInput input int16 size=1; AverageOut output fixdt(1,32,0) size=1; Trigger input boolean size=1; TriggerDelay input uint32 size=1; GateLength input uint16; AveragingFlag output fixdt(0,1,0); DataValid output fixdt(0,1,0)
%auto-generated
%#codegen
function [AverageOut,AveragingFlag,DataValid] = Boxcar_fixpt(SignalInput, Trigger, TriggerDelay, GateLength)

fm = get_fimath();
GateLength = fi(GateLength, 0, 16, 0, fm);
SignalInput = fi(SignalInput, 1, 16, 0, fm);
TriggerDelay = fi(TriggerDelay, 0, 32, 0, fm);

persistent AvgOut;
if isempty(AvgOut)
    AvgOut = fi(0, 1, 32, 0, fm);
end


persistent cnt1;
if isempty(cnt1)
    cnt1 = fi(0, 0, 32, 0, fm);
end

persistent cnt2;
if isempty(cnt2)
    cnt2 = fi(0, 0, 16, 0, fm);
end


persistent AvgFlag;
if isempty(AvgFlag)
    AvgFlag = fi(0, 0, 1, 0, fm);
end

persistent DValid;
if isempty(DValid)
    DValid = fi(0, 0, 1, 0, fm);
end

S1 = fi(0, 0, 2, 0, fm); %Waiting for trigger
S2 = fi(1, 0, 2, 0, fm);
S3 = fi(2, 0, 2, 0, fm);

persistent current_state;
if isempty(current_state)
    current_state = fi(S1, 0, 2, 0, fm);   
end

switch(current_state)

    case S1
        DValid(:) = 0;
        AvgFlag(:) = 0;
        if Trigger == 1
            current_state(:) = S2;
            cnt1(:) = TriggerDelay;
        else
            current_state(:) = S1;
        end

    case S2

        if cnt1 == fi(0, 0, 1, 0, fm)
            current_state(:) = S3;
            cnt2(:) = GateLength;
            AvgOut(:) = 0;
        else
            cnt1(:) = fi_signed(cnt1)-fi(1, 0, 1, 0, fm);
        end

    case S3
        if cnt2 == fi(0, 0, 1, 0, fm)
            current_state(:) = S1;
            DValid(:) = 0;
        else
            AvgOut(:) = AvgOut + SignalInput;
            AvgFlag(:) = 1;
            cnt2(:) = fi_signed(cnt2)-fi(1, 0, 1, 0, fm);
            if cnt2 == fi(0, 0, 1, 0, fm)
                DValid(:) = 1;
                current_state(:) = S1;
            end 
        end

end

AverageOut = fi(AvgOut, 1, 32, 0, fm);
DataValid = fi(DValid, 0, 1, 0, fm);
AveragingFlag = fi(AvgFlag, 0, 1, 0, fm);



end



function y = fi_signed(a)
    coder.inline( 'always' );
    if isfi( a ) && ~(issigned( a ))
        nt = numerictype( a );
        new_nt = numerictype( 1, nt.WordLength + 1, nt.FractionLength );
        y = fi( a, new_nt, fimath( a ) );
    else
        y = a;
    end
end

function fm = get_fimath()
	fm = fimath('RoundingMethod', 'Floor',...
	     'OverflowAction', 'Wrap',...
	     'ProductMode','FullPrecision',...
	     'MaxProductWordLength', 128,...
	     'SumMode','FullPrecision',...
	     'MaxSumWordLength', 128);
end
